simulink model "Rasp_WS"  (R2024b)
settings: Solver=FixedStepAuto  StartTime=0.0  StopTime=inf  RelTol=1e-3  EnableMultiTasking=on
undefined symbols (not defined in the file): Green, led0
libraries: raspberrypiBasiclib x2, raspberrypiCommlib x2, raspberrypiNetworklib x2
settings Model: SimulationMode=external  ExtModeTrigDuration=2  Creator=davil  LastModifiedBy=davil
settings SolverCC: PositivePriorityOrder=on
settings OptimizationCC: DefaultParameterBehavior=Inlined  EnhancedBackFolding=on  PassReuseOutputArgsAs=Individual arguments  ZeroExternalMemoryAtStartup=off  ZeroInternalMemoryAtStartup=off  MaxStackSize=200000  OptimizeBlockOrder=speed  DifferentSizesBufferReuse=on  OptimizationCustomize=off  EfficientTunableParamExpr=on
settings DebuggingCC: ParameterTunabilityLossMsg=error
settings HardwareCC: ProdBitPerPointer=32  ProdBitPerSizeT=32  ProdBitPerPtrDiffT=32  ProdLargestAtomicInteger=Long  ProdLargestAtomicFloat=Double  ProdWordSize=32  ProdLongLongMode=on  ProdHWDeviceType=ARM Compatible->ARM Cortex-A (32-bit)
settings RTWCC: Description=Embedded Coder  SystemTargetFile=ert.tlc  HardwareBoard=Raspberry Pi  TLCOptions="-aInlineSetEventsForThisBaseRateFcn=TLC_FALSE -aSuppressMultiTaskScheduler=TLC_FALSE  -aRateBasedStepFcn=0"  TemplateMakefile=ert_default_tmf  Toolchain=GNU GCC Embedded Linux  BuildConfiguration=Faster Runs
settings CodeAppCC: ForceParamTrailComments=on  IgnoreCustomStorageClasses=off  OperatorAnnotations=on  SimulinkDataObjDesc=on  SFDataObjDesc=on  InsertBlockDesc=on
settings ERTTargetCC: CodeReplacementLibrary=ARM Cortex-A CMSIS  SupportVariableSizeSignals=on  ExtModeTransport=2  ExtModeStaticAlloc=on  ExtModeMexFile=ext_xcp  ExtModeIntrfLevel=Level2 - Open

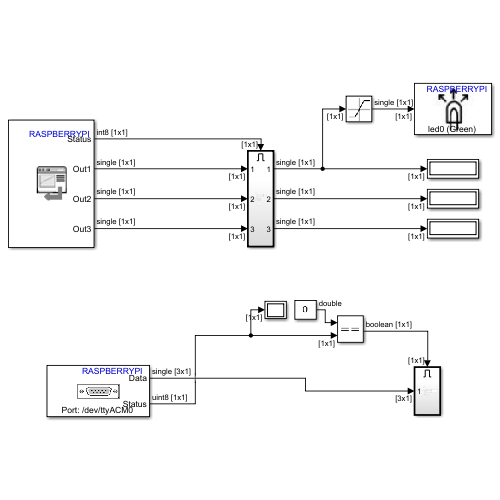
[thumbnail: Simulink's stored preview of the top-level diagram]
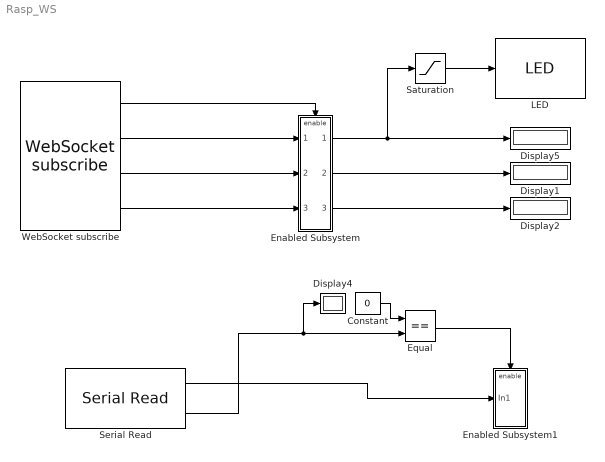
== system Rasp_WS ==
  Constant : Constant  Value=0
  Display{1..2,4..5} (4 alike) : Display
  Enabled Subsystem : Subsystem  TreatAsAtomicUnit=on
  Enabled Subsystem1 : Subsystem  TreatAsAtomicUnit=on
  Equal : RelationalOperator  Operator===  OutDataTypeStr=boolean  RndMeth=Simplest  InputSameDT=off
  LED : raspberrypiBasiclib/LED  BoardProperty=Pi 5 Model  LED_=led0 (Green)
  Saturation : Saturate  UpperLimit=1  LowerLimit=0
  Serial Read : raspberrypiCommlib/Serial Read  board=Pi 5 Model  SCIModule_=/dev/ttyACM0  Baudrate_=9600  Parity=None  StopBits_=1  HardwareFlowControl=None  ByteOrder=LittleEndian  DataLength=3  DataType=single  OutputStatus=on  SampleTime=0.1  blockPlatform=RaspberryPi
  WebSocket subscribe : raspberrypiNetworklib/WebSocket subscribe  IPAddress=172.16.16.134  Port=8080  OutputCfg=Mask Dialog  numSignals=3  Dsize1=1  Dtype1=single  Dsize2=1  Dtype2=single  Dsize3=1  Dtype3=single  Dsize4=1  Dtype4=double  Dsize5=1  Dtype5=double  Dsize6=1  Dtype6=double  Dsize7=1  Dtype7=double  Dsize8=1  Dtype8=double  Dsize9=1  Dtype9=double  Dsize10=1  Dtype10=double  Sampletime=1  NumberOfSignals=3  webSocketId=Rasp_WS/WebSocket_subscribe  BlockPlatform=RASPBERRYPI
  wires:
  WebSocket subscribe/1 -> Enabled Subsystem/Enable
  WebSocket subscribe/3 -> Enabled Subsystem/2(In2)
  Enabled Subsystem/2(Out2) -> Display1/1
  WebSocket subscribe/2 -> Enabled Subsystem/1(In1)
  Enabled Subsystem/1(Out1) -> Display5/1, Saturation/1
  Saturation/1 -> LED/1
  WebSocket subscribe/4 -> Enabled Subsystem/3(In3)
  Enabled Subsystem/3(Out3) -> Display2/1
  Constant/1 -> Equal/1
  Equal/1 -> Enabled Subsystem1/Enable
  Serial Read/2 -> Display4/1, Equal/2
  Serial Read/1 -> Enabled Subsystem1/1(In1)

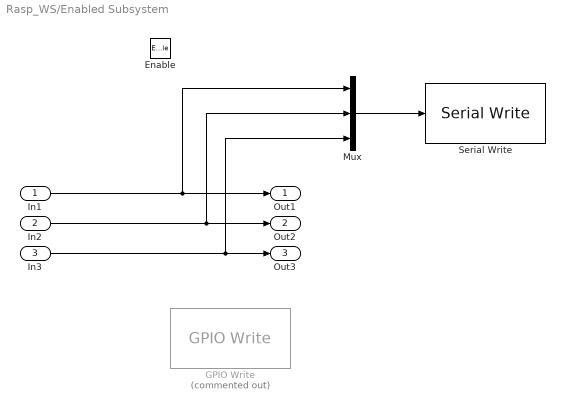
== system Rasp_WS/Enabled Subsystem ==
  In1 : Inport
  In2 : Inport  Port=2
  In3 : Inport  Port=3
  Enable : EnablePort
  GPIO Write : raspberrypiBasiclib/GPIO Write  Commented=on  BoardProperty=Pi 5 Model  gpio=2  blockPlatform=Raspberry Pi  PinNumber=17  board=[]  direction=[]
  Mux : Mux  Inputs=3
  Serial Write : raspberrypiCommlib/Serial Write  board=Pi 5 Model  SCIModule_=/dev/ttyACM0  Baudrate_=9600  Parity=None  StopBits_=1  HardwareFlowControl=None  ByteOrder=LittleEndian  OutputStatus=off  blockPlatform=RaspberryPi
  Out1 : Outport
  Out2 : Outport  Port=2
  Out3 : Outport  Port=3
  wires:
  In2/1 -> Mux/2, Out2/1
  In3/1 -> Mux/3, Out3/1
  In1/1 -> Mux/1, Out1/1
  Mux/1 -> Serial Write/1

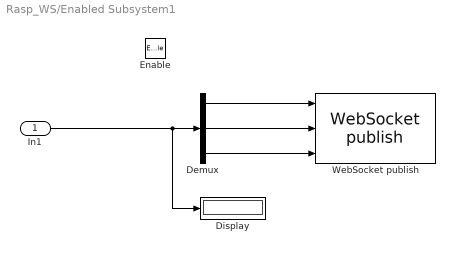
== system Rasp_WS/Enabled Subsystem1 ==
  In1 : Inport
  Enable : EnablePort
  Demux : Demux  Outputs=3
  Display : Display
  WebSocket publish : raspberrypiNetworklib/WebSocket publish  UniqueBlockID=webPub 1  IPAddress=172.16.16.134  Port=8080  NumberOfSignals=3  webSocketId=Rasp_WS/Enabled_Subsystem1/WebSocket_publish  BlockPlatform=RASPBERRYPI
  wires:
  In1/1 -> Display/1, Demux/1
  Demux/2 -> WebSocket publish/2
  Demux/1 -> WebSocket publish/1
  Demux/3 -> WebSocket publish/3
